simulink model "bldc_motor_model"  (R2020b)
settings: Solver=VariableStepAuto  StartTime=0.0  StopTime=10  RelTol=1e-3
values from neighbouring files (symbols this model uses):
  Ke = 0.01    [model_paramtrs.sldd]
  L = 0.5    [model_paramtrs.sldd]
  R = 1.0    [model_paramtrs.sldd]
undefined symbols (not defined in the file or in its folder): B, J, Kt
libraries: pid_lib x1
settings Model: DataDictionary=model_paramtrs.sldd  Creator=153  LastModifiedBy=153

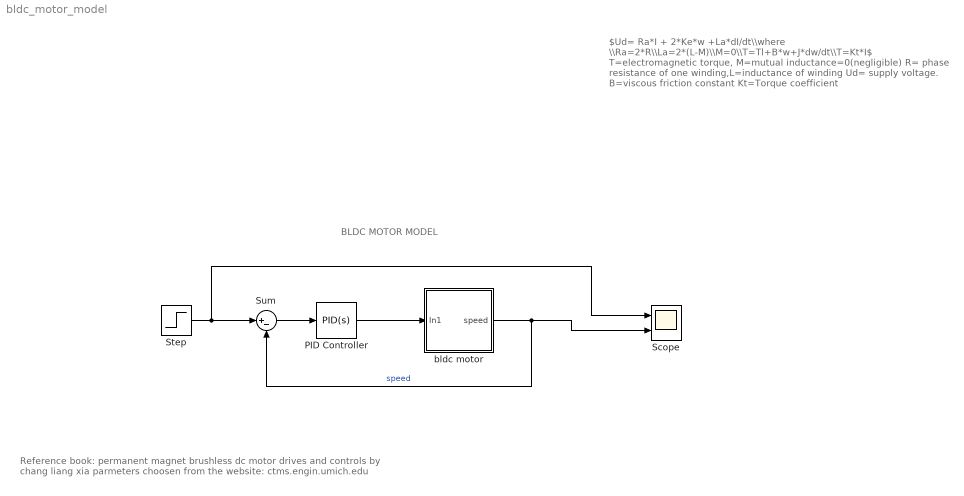
== system bldc_motor_model ==
  note: $Ud= Ra*I + 2*Ke*w +La*dI/dt\\where \\Ra=2*R\\La=2*(L-M)\\M=0\\T=Tl+B*w+J*dw/dt\\T=Kt*I$
      |
      | T=electromagnetic torque, M=mutual inductance=0(negligible)
      | R= phase resistance of one winding,L=inductance of winding
      | Ud= supply voltage. B=viscous friction constant Kt=Torque coefficient
  note: Reference book: permanent magnet brushless dc motor drives and controls
      | by chang liang xia
      |  parmeters choosen from the website: ctms.engin.umich.edu
  note: BLDC MOTOR MODEL
  PID Controller : pid_lib/PID Controller  Controller=PID  Form=Parallel  TimeDomain=Continuous-time  UseExternalTs=off  SampleTime=-1  IntegratorMethod=Forward Euler  FilterMethod=Forward Euler  ControllerParametersSource=internal  P=165  I=105  D=1  UseFilter=on  N=100  TunerSelectOption=Transfer Function Based (PID Tuner App)  InitialConditionSource=internal  InitialConditionForIntegrator=0  InitialConditionForFilter=0  DifferentiatorICPrevScaledInput=0  ExternalReset=none  TrackingMode=off  Kt=1  LimitOutput=off  SatLimitsSource=internal  UpperSaturationLimit=inf  LowerSaturationLimit=-inf  LinearizeAsGain=on  AntiWindupMode=none  Kb=1  POutMin=[]  POutMax=[]  IOutMin=[]  IOutMax=[]  DOutMin=[]  DOutMax=[]  NOutMin=[]  NOutMax=[]  SumOutMin=[]  SumOutMax=[]  SaturationOutMin=[]  SaturationOutMax=[]  PParamMin=[]  PParamMax=[]  IParamMin=[]  IParamMax=[]  DParamMin=[]  DParamMax=[]  NParamMin=[]  NParamMax=[]  KbParamMin=[]  KbParamMax=[]  KtParamMin=[]  KtParamMax=[]  KbOutMin=[]  KbOutMax=[]  KtOutMin=[]  KtOutMax=[]  IntegratorOutMin=[]  IntegratorOutMax=[]  FilterOutMin=[]  FilterOutMax=[]  SumI1OutMin=[]  SumI1OutMax=[]  SumI2OutMin=[]  SumI2OutMax=[]  SumI3OutMin=[]  SumI3OutMax=[]  SumI4OutMin=[]  SumI4OutMax=[]  SumDOutMin=[]  SumDOutMax=[]  DifferentiatorOutMin=[]  DifferentiatorOutMax=[]  FilterDiffOutCoefMin=[]  FilterDiffOutCoefMax=[]  ReciprocalOutMin=[]  ReciprocalOutMax=[]  SumDenOutMin=[]  SumDenOutMax=[]  SumNumOutMin=[]  SumNumOutMax=[]  DivideOutMin=[]  DivideOutMax=[]  UdiffTsProdOutMin=[]  UdiffTsProdOutMax=[]  NTsProdOutMin=[]  NTsProdOutMax=[]  UintegralTsProdOutMin=[]  UintegralTsProdOutMax=[]  UngainTsProdOutMin=[]  UngainTsProdOutMax=[]  IntegratorContinuousStateAttributes=''  IntegratorStateMustResolveToSignalObject=off  IntegratorRTWStateStorageClass=Auto  FilterContinuousStateAttributes=''  FilterStateMustResolveToSignalObject=off  FilterRTWStateStorageClass=Auto  ParallelPVariant=InternalParameters  IdealPVariant=Disabled  IVariant=InternalParameters  DVariant=InternalParameters  IntegratorVariant=Continuous  SatVariant=Disabled  AWVariant=Passthrough  PCopyVariant=Disabled  TRVariant=Disabled  FdbkBlocksVariant=Forward  IdealPFdbkVariant=Disabled  SatFdbkVariant=Disabled  DerivativeFilterVariant=ContFilter  NVariant=InternalParameters  NCopyVariant=Disabled  FilterICVariant=InternalICsFilter  IntegratorICVariant=InternalICs  ExternalResetVariant=Disabled  TRSumVariant=Passthrough  SumFdbkVariant=Disabled  SumVariant=Sum_PID  TsampFilterVariant=InternalTs  TsampNgainVariant=Passthrough  TsampIntegralVariant=Passthrough  ExternalSaturationOutDataTypeStr=Inherit: Same as second input
  Scope : Scope  NumInputPorts=2
  Step : Step  SampleTime=0
  Sum : Sum  Inputs=|+-
  bldc motor : Subsystem
  wires:
  bldc motor/1(speed) -> Sum/2, Scope/2  "speed"
  Step/1 -> Sum/1, Scope/1
  PID Controller/1 -> bldc motor/1(In1)
  Sum/1 -> PID Controller/1

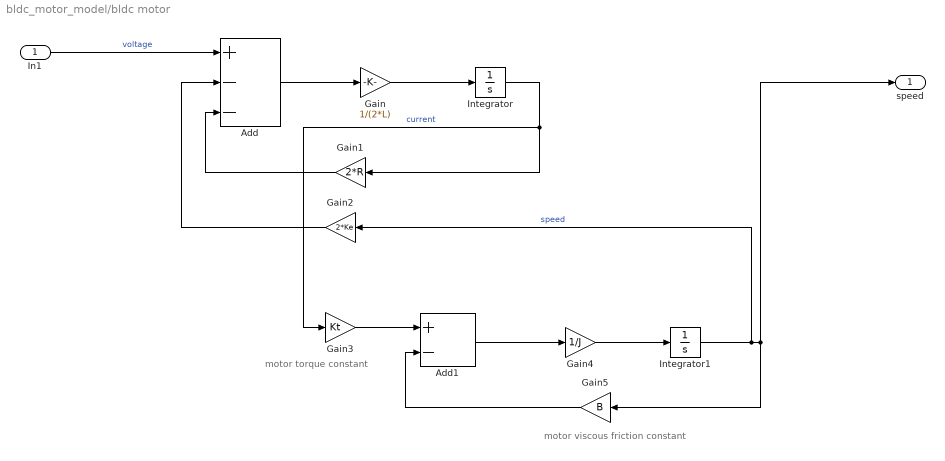
== system bldc_motor_model/bldc motor ==
  note: motor viscous friction constant
  note: motor torque constant
  In1 : Inport
  Add : Sum  Inputs=+--
  Add1 : Sum  Inputs=+-
  Gain : Gain  Gain=1/(2*L)
  Gain1 : Gain  Gain=2*R
  Gain2 : Gain  Gain=2*Ke
  Gain3 : Gain  Gain=Kt
  Gain4 : Gain  Gain=1/J
  Gain5 : Gain  Gain=B
  Integrator : Integrator
  Integrator1 : Integrator
  speed : Outport
  wires:
  Add1/1 -> Gain4/1
  Gain/1 -> Integrator/1
  Integrator1/1 -> Gain2/1, speed/1, Gain5/1  "speed"
  Integrator/1 -> Gain1/1, Gain3/1  "current"
  Gain4/1 -> Integrator1/1
  Gain1/1 -> Add/3
  Add/1 -> Gain/1
  Gain5/1 -> Add1/2
  Gain3/1 -> Add1/1
  Gain2/1 -> Add/2
  In1/1 -> Add/1  "voltage"
